simulink model "aae364gantry2"  (Simulink 10.3)
settings: Solver=ode4  StartTime=0.0  StopTime=80  FixedStep=0.002  RelTol=1e-3  AbsTol=1e-6
values from neighbouring files (symbols this model uses):
  Beq = 5.4    [setup_ip01_2_configuration.m]
  Bp = 0.0024    [setup_sp_configuration.m]
  Eff_g = 1    [setup_ip01_2_configuration.m]
  Eff_m = 1    [setup_ip01_2_configuration.m]
  g = 9.81    [setup_sp_configuration.m]
  IMAX_UPM = 3    [setup_ip01_2_configuration.m]
  Ip = Mp * Lp^2 / 12    [setup_sp_configuration.m]
  K = place( A, B, cl_poles )    [d_ip02_spg_pp.m]    (also in setup_lab_ip02_spg.m = [ 0 0 0 0 ])
  Kg = 3.71    [setup_ip01_2_configuration.m]
  Km = 0.804e-3 * K_RDPS2RPM    [setup_ip01_2_configuration.m]
  Kt = 1.088 * K_OZ2N * K_IN2M    [setup_ip01_2_configuration.m]
  lp = 7 * K_IN2M    [setup_sp_configuration.m]
  Mc = Mc + Eff_g * Kg^2 * Jm / r_mp^2    [setup_lab_ip02_spg.m]
  Mp = 0.127    [setup_sp_configuration.m]
  r_mp = 0.5 / 2 * K_IN2M    [setup_ip01_2_configuration.m]
  Rm = 2.6    [setup_ip01_2_configuration.m]
  VMAX_UPM = 13    [setup_ip01_2_configuration.m]
  X0 = [ 0; X0(2); 0; 0 ]    [setup_lab_ip02_spg.m]
libraries: simulink x1
settings Model: Creator=art  LastModifiedBy=Joseph  ExtModeArmWhenConnect=off  ExtModeAutoUpdateStatusClock=off
settings SolverCC: AutoScaleAbsTol=off
settings OptimizationCC: BooleanDataType=off  OptimizeBlockIOStorage=off  BufferReuse=off  ExpressionFolding=off  LocalBlockOutputs=off  InitFltsAndDblsToZero=on
settings DebuggingCC: SaveWithParameterizedLinksMsg=none  SignalResolutionControl=TryResolveAllWithWarning  MultiTaskDSMMsg=warning  MultiTaskCondExecSysMsg=none
settings HardwareCC: TargetUnknown=on
settings RTWCC: SystemTargetFile=wincon.tlc  MakeCommand=make_wc  TemplateMakefile=nt_msvc.tmf
settings STFCustomTargetCC: TargetFcnLib=ansi_tfl_tmw.mat  ModelReferenceCompliant=off  CPPClassGenCompliant=on  SystemTargetFile=wincon.tlc
settings GRTTargetCC: TargetFcnLib=ansi_tfl_tmw.mat  ModelReferenceCompliant=off  ParMdlRefBuildCompliant=off  CompOptLevelCompliant=off  ConcurrentExecutionCompliant=off  MatFileLogging=off  UseToolchainInfoCompliant=off  ExtModeMexFile=noextcomm
settings CustomProperty: Value=on

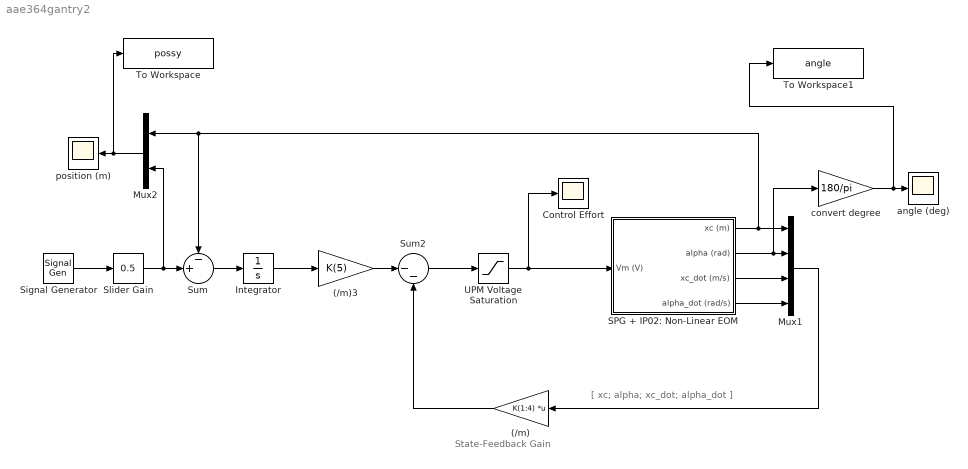
== system aae364gantry2 ==
  note: [ xc; alpha; xc_dot; alpha_dot ]
  note: State-Feedback Gain
  (/m) : Gain  Gain=K(1:4)  Multiplication=Matrix(K*u)  SaturateOnIntegerOverflow=on  OutDataTypeStr=Inherit: Same as input  ParamDataTypeStr=Inherit: Same as input
  (/m)3 : Gain  Gain=K(5)  SaturateOnIntegerOverflow=on  OutDataTypeStr=Inherit: Same as input  ParamDataTypeStr=Inherit: Same as input
  Control Effort : Scope
  Integrator : Integrator
  Mux1 : Mux
  Mux2 : Mux  Inputs=2
  SPG + IP02: Non-Linear EOM : Subsystem
  Signal Generator : SignalGenerator  WaveForm=square  Amplitude=.5  Frequency=.1
  Slider Gain : simulink/Math Operations/Slider Gain  gain=0.5  low=0  high=2
  Sum : Sum  Inputs=-+|
  Sum2 : Sum  Inputs=|--  InputSameDT=on  SaturateOnIntegerOverflow=on  OutDataTypeStr=Inherit: Same as first input
  To Workspace : ToWorkspace  VariableName=possy  SaveFormat=Timeseries  SampleTime=-1
  To Workspace1 : ToWorkspace  VariableName=angle  SaveFormat=Timeseries  SampleTime=-1
  UPM Voltage Saturation : Saturate  UpperLimit=VMAX_UPM  LowerLimit=- VMAX_UPM
  angle (deg) : Scope
  convert degree : Gain  Gain=180/pi
  position (m) : Scope
  wires:
  UPM Voltage Saturation/1 -> Control Effort/1, SPG + IP02: Non-Linear EOM/1(Vm (V))
  (/m)3/1 -> Sum2/1
  Sum/1 -> Integrator/1
  Mux1/1 -> (/m)/1
  (/m)/1 -> Sum2/2
  SPG + IP02: Non-Linear EOM/2(alpha (rad)) -> Mux1/2, convert degree/1
  SPG + IP02: Non-Linear EOM/3(xc_dot (m/s)) -> Mux1/3
  SPG + IP02: Non-Linear EOM/4(alpha_dot (rad/s)) -> Mux1/4
  Sum2/1 -> UPM Voltage Saturation/1
  Integrator/1 -> (/m)3/1
  Signal Generator/1 -> Slider Gain/1
  SPG + IP02: Non-Linear EOM/1(xc (m)) -> Mux1/1, Sum/1, Mux2/1
  convert degree/1 -> To Workspace1/1, angle (deg)/1
  Slider Gain/1 -> Sum/2, Mux2/2
  Mux2/1 -> To Workspace/1, position (m)/1

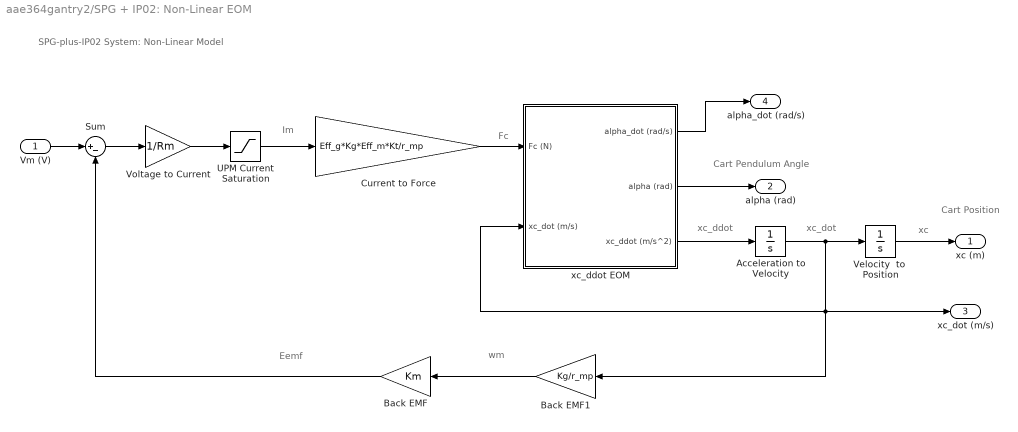
== system aae364gantry2/SPG + IP02: Non-Linear EOM ==
  note: SPG-plus-IP02 System:
      | Non-Linear Model
  note: Fc
  note: Im
  note: Eemf
  note: wm
  note: xc_dot
  note: xc_ddot
  note: xc
  note: Cart Position
  note: Cart Pendulum Angle
  Vm (V) : Inport
  Acceleration to Velocity : Integrator
  Back EMF : Gain  Gain=Km  SaturateOnIntegerOverflow=on  OutDataTypeStr=Inherit: Same as input  ParamDataTypeStr=Inherit: Same as input
  Back EMF1 : Gain  Gain=Kg/r_mp  SaturateOnIntegerOverflow=on  OutDataTypeStr=Inherit: Same as input  ParamDataTypeStr=Inherit: Same as input
  Current to Force : Gain  Gain=Eff_g*Kg*Eff_m*Kt/r_mp  SaturateOnIntegerOverflow=on  OutDataTypeStr=Inherit: Same as input  ParamDataTypeStr=Inherit: Same as input
  Sum : Sum  Inputs=|+-  InputSameDT=on  SaturateOnIntegerOverflow=on  OutDataTypeStr=Inherit: Same as first input
  "UPM Current Saturation " : Saturate  UpperLimit=IMAX_UPM  LowerLimit=- IMAX_UPM
  Velocity  to  Position : Integrator
  Voltage to Current : Gain  Gain=1/Rm  SaturateOnIntegerOverflow=on  OutDataTypeStr=Inherit: Same as input  ParamDataTypeStr=Inherit: Same as input
  xc_ddot EOM : Subsystem
  xc (m) : Outport
  alpha (rad) : Outport  Port=2
  xc_dot (m/s) : Outport  Port=3  InitialOutput=0
  alpha_dot (rad/s) : Outport  Port=4  InitialOutput=0
  wires:
  Sum/1 -> Voltage to Current/1
  Voltage to Current/1 -> "UPM Current Saturation "/1
  Acceleration to Velocity/1 -> xc_dot (m/s)/1, Back EMF1/1, xc_ddot EOM/2(xc_dot (m/s)), Velocity  to  Position/1
  Back EMF1/1 -> Back EMF/1
  Vm (V)/1 -> Sum/1
  Velocity  to  Position/1 -> xc (m)/1
  Back EMF/1 -> Sum/2
  "UPM Current Saturation "/1 -> Current to Force/1
  Current to Force/1 -> xc_ddot EOM/1(Fc (N))
  xc_ddot EOM/3(xc_ddot (m/s^2)) -> Acceleration to Velocity/1
  xc_ddot EOM/2(alpha (rad)) -> alpha (rad)/1
  xc_ddot EOM/1(alpha_dot (rad/s)) -> alpha_dot (rad/s)/1

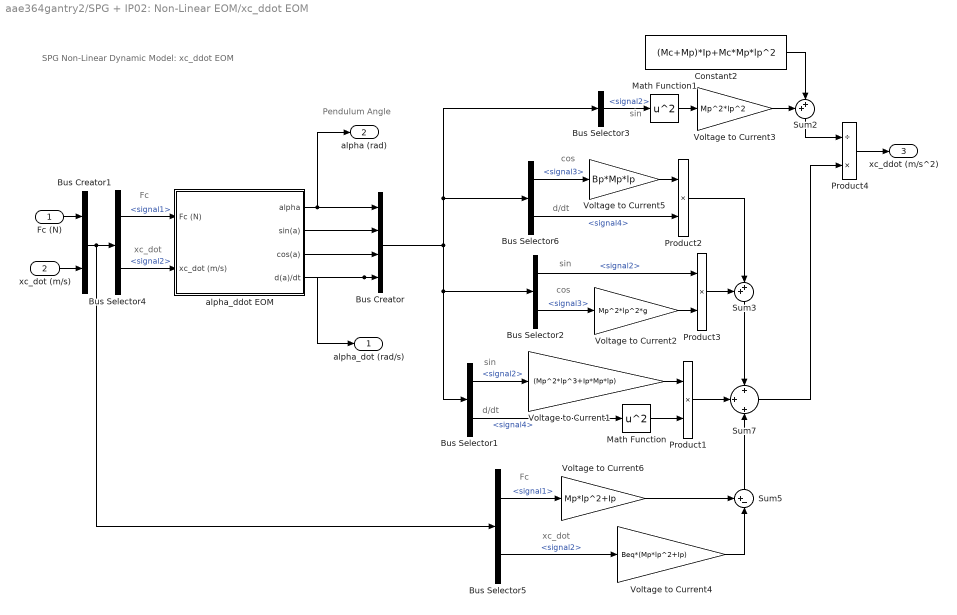
== system aae364gantry2/SPG + IP02: Non-Linear EOM/xc_ddot EOM ==
  note: d/dt
  note: sin
  note: sin
  note: cos
  note: sin
  note: Pendulum Angle
  note: cos
  note: d/dt
  note: Fc
  note: xc_dot
  note: Fc
  note: xc_dot
  note: SPG Non-Linear Dynamic Model:
      | xc_ddot EOM
  Fc (N) : Inport
  xc_dot (m/s) : Inport  Port=2
  Bus Creator : BusCreator  Inputs=4
  Bus Creator1 : BusCreator  Inputs=2
  Bus Selector1 : BusSelector  OutputSignals=signal2,signal4
  Bus Selector2 : BusSelector  OutputSignals=signal2,signal3
  Bus Selector3 : BusSelector  OutputSignals=signal2
  Bus Selector4 : BusSelector  OutputSignals=signal1,signal2
  Bus Selector5 : BusSelector  OutputSignals=signal1,signal2
  Bus Selector6 : BusSelector  OutputSignals=signal3,signal4
  Constant2 : Constant  Value=(Mc+Mp)*Ip+Mc*Mp*lp^2
  Math Function : Math  Operator=square  SignedPower=on  SaturateOnIntegerOverflow=on
  Math Function1 : Math  Operator=square  SignedPower=on  SaturateOnIntegerOverflow=on
  Product1 : Product  InputSameDT=on  RndMeth=Zero  SaturateOnIntegerOverflow=on  OutDataTypeStr=Inherit: Same as first input
  Product2 : Product  InputSameDT=on  RndMeth=Zero  SaturateOnIntegerOverflow=on  OutDataTypeStr=Inherit: Same as first input
  Product3 : Product  InputSameDT=on  RndMeth=Zero  SaturateOnIntegerOverflow=on  OutDataTypeStr=Inherit: Same as first input
  Product4 : Product  Inputs=/*  InputSameDT=on  RndMeth=Zero  SaturateOnIntegerOverflow=on  OutDataTypeStr=Inherit: Same as first input
  Sum2 : Sum  Inputs=++|  InputSameDT=on  SaturateOnIntegerOverflow=on  OutDataTypeStr=Inherit: Same as first input
  Sum3 : Sum  Inputs=++|  InputSameDT=on  SaturateOnIntegerOverflow=on  OutDataTypeStr=Inherit: Same as first input
  Sum5 : Sum  Inputs=+-|  InputSameDT=on  SaturateOnIntegerOverflow=on  OutDataTypeStr=Inherit: Same as first input
  Sum7 : Sum  Inputs=+|+|+  InputSameDT=on  SaturateOnIntegerOverflow=on  OutDataTypeStr=Inherit: Same as first input
  Voltage to Current1 : Gain  Gain=(Mp^2*lp^3+Ip*Mp*lp)  SaturateOnIntegerOverflow=on  OutDataTypeStr=Inherit: Same as input  ParamDataTypeStr=Inherit: Same as input
  Voltage to Current2 : Gain  Gain=Mp^2*lp^2*g  SaturateOnIntegerOverflow=on  OutDataTypeStr=Inherit: Same as input  ParamDataTypeStr=Inherit: Same as input
  Voltage to Current3 : Gain  Gain=Mp^2*lp^2  SaturateOnIntegerOverflow=on  OutDataTypeStr=Inherit: Same as input  ParamDataTypeStr=Inherit: Same as input
  Voltage to Current4 : Gain  Gain=Beq*(Mp*lp^2+Ip)  SaturateOnIntegerOverflow=on  OutDataTypeStr=Inherit: Same as input  ParamDataTypeStr=Inherit: Same as input
  Voltage to Current5 : Gain  Gain=Bp*Mp*lp  SaturateOnIntegerOverflow=on  OutDataTypeStr=Inherit: Same as input  ParamDataTypeStr=Inherit: Same as input
  Voltage to Current6 : Gain  Gain=Mp*lp^2+Ip  SaturateOnIntegerOverflow=on  OutDataTypeStr=Inherit: Same as input  ParamDataTypeStr=Inherit: Same as input
  alpha_ddot EOM : Subsystem
  alpha_dot (rad/s) : Outport
  alpha (rad) : Outport  Port=2
  xc_ddot (m/s^2) : Outport  Port=3
  wires:
  Sum2/1 -> Product4/1
  Bus Creator/1 -> Bus Selector2/1, Bus Selector1/1, Bus Selector3/1, Bus Selector6/1
  Voltage to Current1/1 -> Product1/1
  Math Function/1 -> Product1/2
  Voltage to Current2/1 -> Product3/2
  Bus Selector3/1 -> Math Function1/1  "<signal2>"
  Math Function1/1 -> Voltage to Current3/1
  Voltage to Current3/1 -> Sum2/1
  Constant2/1 -> Sum2/2
  Product1/1 -> Sum7/2
  Product4/1 -> xc_ddot (m/s^2)/1
  alpha_ddot EOM/1(alpha) -> Bus Creator/1, alpha (rad)/1
  alpha_ddot EOM/2(sin(a)) -> Bus Creator/2
  alpha_ddot EOM/3(cos(a)) -> Bus Creator/3
  alpha_ddot EOM/4(d(a)/dt) -> Bus Creator/4, alpha_dot (rad/s)/1
  Fc (N)/1 -> Bus Creator1/1
  xc_dot (m/s)/1 -> Bus Creator1/2
  Bus Creator1/1 -> Bus Selector4/1, Bus Selector5/1
  Bus Selector4/1 -> alpha_ddot EOM/1(Fc (N))  "<signal1>"
  Bus Selector4/2 -> alpha_ddot EOM/2(xc_dot (m/s))  "<signal2>"
  Bus Selector1/2 -> Math Function/1  "<signal4>"
  Bus Selector1/1 -> Voltage to Current1/1  "<signal2>"
  Bus Selector6/1 -> Voltage to Current5/1  "<signal3>"
  Bus Selector6/2 -> Product2/2  "<signal4>"
  Bus Selector2/1 -> Product3/1  "<signal2>"
  Bus Selector2/2 -> Voltage to Current2/1  "<signal3>"
  Voltage to Current5/1 -> Product2/1
  Bus Selector5/1 -> Voltage to Current6/1  "<signal1>"
  Bus Selector5/2 -> Voltage to Current4/1  "<signal2>"
  Sum7/1 -> Product4/2
  Product2/1 -> Sum3/2
  Product3/1 -> Sum3/1
  Sum3/1 -> Sum7/1
  Sum5/1 -> Sum7/3
  Voltage to Current6/1 -> Sum5/1
  Voltage to Current4/1 -> Sum5/2

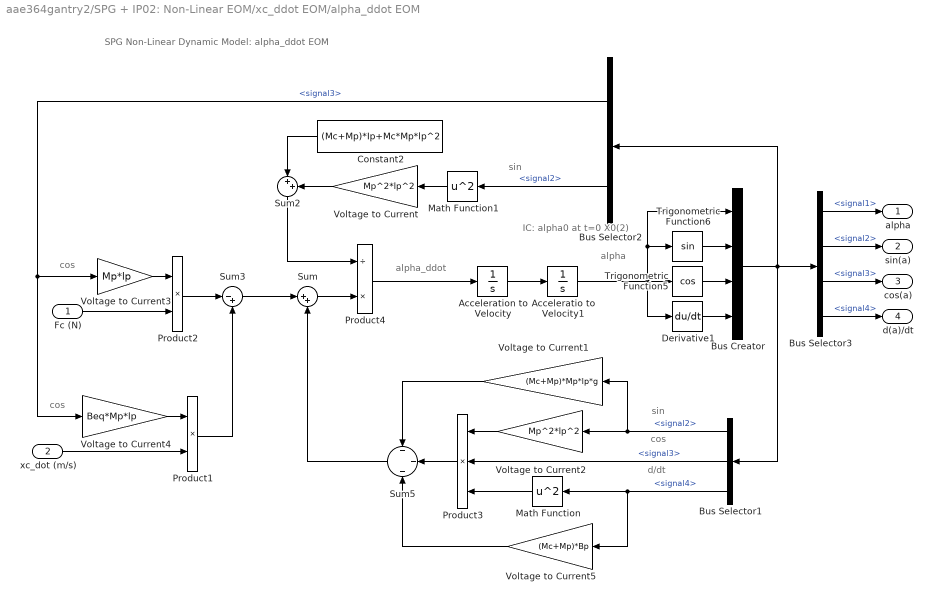
== system aae364gantry2/SPG + IP02: Non-Linear EOM/xc_ddot EOM/alpha_ddot EOM ==
  note: d/dt
  note: cos
  note: sin
  note: cos
  note: sin
  note: alpha
  note: IC: alpha0 at t=0
      | X0(2)
  note: alpha_ddot
  note: cos
  note: SPG Non-Linear Dynamic Model:
      | alpha_ddot EOM
  Fc (N) : Inport
  xc_dot (m/s) : Inport  Port=2
  Acceleratio to Velocity1 : Integrator  InitialCondition=X0(2)
  Acceleration to Velocity : Integrator
  Bus Creator : BusCreator  Inputs=4
  Bus Selector1 : BusSelector  OutputSignals=signal2,signal3,signal4
  Bus Selector2 : BusSelector  OutputSignals=signal3,signal2
  Bus Selector3 : BusSelector  OutputSignals=signal1,signal2,signal3,signal4
  Constant2 : Constant  Value=(Mc+Mp)*Ip+Mc*Mp*lp^2
  Derivative1 : Derivative
  Math Function : Math  Operator=square  SignedPower=on  SaturateOnIntegerOverflow=on
  Math Function1 : Math  Operator=square  SignedPower=on  SaturateOnIntegerOverflow=on
  Product1 : Product  InputSameDT=on  RndMeth=Zero  SaturateOnIntegerOverflow=on  OutDataTypeStr=Inherit: Same as first input
  Product2 : Product  InputSameDT=on  RndMeth=Zero  SaturateOnIntegerOverflow=on  OutDataTypeStr=Inherit: Same as first input
  Product3 : Product  Inputs=3  InputSameDT=on  RndMeth=Zero  SaturateOnIntegerOverflow=on  OutDataTypeStr=Inherit: Same as first input
  Product4 : Product  Inputs=/*  InputSameDT=on  RndMeth=Zero  SaturateOnIntegerOverflow=on  OutDataTypeStr=Inherit: Same as first input
  Sum : Sum  Inputs=|++  InputSameDT=on  SaturateOnIntegerOverflow=on  OutDataTypeStr=Inherit: Same as first input
  Sum2 : Sum  Inputs=|++  InputSameDT=on  SaturateOnIntegerOverflow=on  OutDataTypeStr=Inherit: Same as first input
  Sum3 : Sum  Inputs=|-+  InputSameDT=on  SaturateOnIntegerOverflow=on  OutDataTypeStr=Inherit: Same as first input
  Sum5 : Sum  Inputs=-|-|-  InputSameDT=on  SaturateOnIntegerOverflow=on  OutDataTypeStr=Inherit: Same as first input
  Trigonometric Function5 : Trigonometry  Operator=cos
  Trigonometric Function6 : Trigonometry
  Voltage to Current : Gain  Gain=Mp^2*lp^2  SaturateOnIntegerOverflow=on  OutDataTypeStr=Inherit: Same as input  ParamDataTypeStr=Inherit: Same as input
  Voltage to Current1 : Gain  Gain=(Mc+Mp)*Mp*lp*g  SaturateOnIntegerOverflow=on  OutDataTypeStr=Inherit: Same as input  ParamDataTypeStr=Inherit: Same as input
  Voltage to Current2 : Gain  Gain=Mp^2*lp^2  SaturateOnIntegerOverflow=on  OutDataTypeStr=Inherit: Same as input  ParamDataTypeStr=Inherit: Same as input
  Voltage to Current3 : Gain  Gain=Mp*lp  SaturateOnIntegerOverflow=on  OutDataTypeStr=Inherit: Same as input  ParamDataTypeStr=Inherit: Same as input
  Voltage to Current4 : Gain  Gain=Beq*Mp*lp  SaturateOnIntegerOverflow=on  OutDataTypeStr=Inherit: Same as input  ParamDataTypeStr=Inherit: Same as input
  Voltage to Current5 : Gain  Gain=(Mc+Mp)*Bp  SaturateOnIntegerOverflow=on  OutDataTypeStr=Inherit: Same as input  ParamDataTypeStr=Inherit: Same as input
  alpha : Outport  InitialOutput=0
  sin(a) : Outport  Port=2  InitialOutput=0
  cos(a) : Outport  Port=3  InitialOutput=0
  d(a)/dt : Outport  Port=4  InitialOutput=0
  wires:
  Acceleration to Velocity/1 -> Acceleratio to Velocity1/1
  Bus Selector1/1 -> Voltage to Current1/1, Voltage to Current2/1  "<signal2>"
  Product4/1 -> Acceleration to Velocity/1
  Math Function/1 -> Product3/3
  Sum2/1 -> Product4/1
  Sum/1 -> Product4/2
  Voltage to Current/1 -> Sum2/2
  Bus Selector2/2 -> Math Function1/1  "<signal2>"
  Math Function1/1 -> Voltage to Current/1
  Constant2/1 -> Sum2/1
  Trigonometric Function6/1 -> Bus Creator/2
  Trigonometric Function5/1 -> Bus Creator/3
  Derivative1/1 -> Bus Creator/4
  Bus Creator/1 -> Bus Selector2/1, Bus Selector1/1, Bus Selector3/1
  Bus Selector2/1 -> Voltage to Current3/1, Voltage to Current4/1  "<signal3>"
  Voltage to Current2/1 -> Product3/1
  Bus Selector1/2 -> Product3/2  "<signal3>"
  Bus Selector1/3 -> Math Function/1, Voltage to Current5/1  "<signal4>"
  Bus Selector3/1 -> alpha/1  "<signal1>"
  Bus Selector3/2 -> sin(a)/1  "<signal2>"
  Bus Selector3/3 -> cos(a)/1  "<signal3>"
  Bus Selector3/4 -> d(a)/dt/1  "<signal4>"
  Acceleratio to Velocity1/1 -> Trigonometric Function5/1, Derivative1/1, Trigonometric Function6/1, Bus Creator/1
  Voltage to Current3/1 -> Product2/1
  Fc (N)/1 -> Product2/2
  xc_dot (m/s)/1 -> Product1/2
  Voltage to Current4/1 -> Product1/1
  Product2/1 -> Sum3/1
  Product1/1 -> Sum3/2
  Sum3/1 -> Sum/1
  Product3/1 -> Sum5/2
  Voltage to Current1/1 -> Sum5/1
  Voltage to Current5/1 -> Sum5/3
  Sum5/1 -> Sum/2
